simulink model "sim_dinamica_completa_pd"  (R2019b)
settings: Solver=VariableStepAuto  StartTime=0.0  StopTime=10  FixedStep=0.01  RelTol=1e-6
values from neighbouring files (symbols this model uses):
  Kd = [Kp1*Td1 0;         0       Kp2*Td2]    [control_pd_g.m]
  Kp = [Kp1 0;         0   Kp2]    [control_pd_g.m]
  q0 = [90*pi/180;0;0;0]    [control_pd_g.m]
  q_ = [110*pi/180;-30*pi/180;0;0]    [control_pd_g.m]
  theta = load('../theta.mat').theta    [control_pd_g.m]    (also in modelo_dinamico_lineal.m)
settings Model: Creator=AlejnadroZapett  LastModifiedBy=AlejnadroZapett

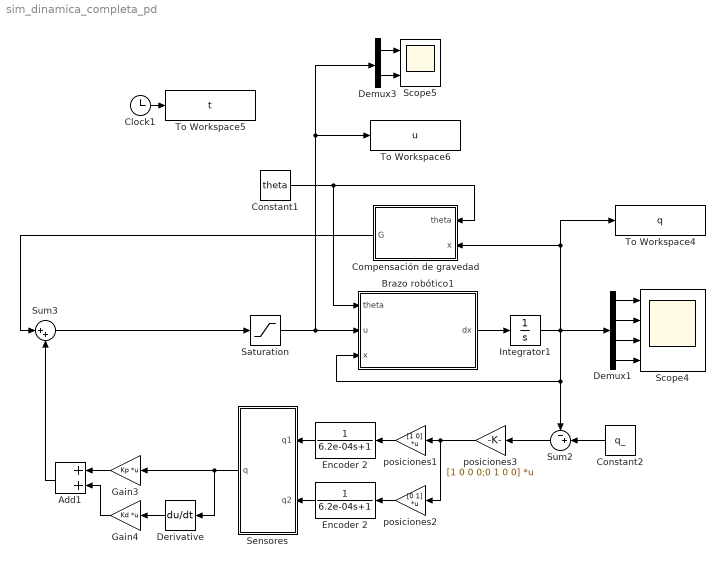
== system sim_dinamica_completa_pd ==
  " Encoder 2 " : TransferFcn  Denominator=[6.2e-04 1]
  Add1 : Sum
  Brazo robótico1 : MATLAB Function  TreatAsAtomicUnit=on
  Clock1 : Clock
  Compensación de gravedad : MATLAB Function  TreatAsAtomicUnit=on
  Constant1 : Constant  Value=theta
  Constant2 : Constant  Value=q_
  Demux1 : Demux
  Demux3 : Demux  Outputs=2
  Derivative : Derivative
  Encoder 2 : TransferFcn  Denominator=[6.2e-04 1]
  Gain3 : Gain  Gain=Kp  Multiplication=Matrix(K*u) (u vector)
  Gain4 : Gain  Gain=Kd  Multiplication=Matrix(K*u) (u vector)
  Integrator1 : Integrator  InitialCondition=q0
  Saturation : Saturate  UpperLimit=255  LowerLimit=-255
  Scope4 : Scope  NumInputPorts=4
  Scope5 : Scope  NumInputPorts=2
  Sensores : MATLAB Function  TreatAsAtomicUnit=on
  Sum2 : Sum  Inputs=-+|
  Sum3 : Sum  Inputs=|++
  To Workspace4 : ToWorkspace  VariableName=q  SampleTime=-1
  To Workspace5 : ToWorkspace  VariableName=t  SampleTime=-1
  To Workspace6 : ToWorkspace  VariableName=u  SampleTime=-1
  posiciones1 : Gain  Gain=[1 0]  Multiplication=Matrix(K*u) (u vector)
  posiciones2 : Gain  Gain=[0 1]  Multiplication=Matrix(K*u) (u vector)
  posiciones3 : Gain  Gain=[1 0 0 0;0 1 0 0]  Multiplication=Matrix(K*u) (u vector)
  wires:
  posiciones2/1 -> Encoder 2/1
  posiciones1/1 -> " Encoder 2 "/1
  Sum2/1 -> posiciones3/1
  Add1/1 -> Sum3/2
  Demux1/4 -> Scope4/4
  Constant2/1 -> Sum2/2
  Demux3/1 -> Scope5/1
  Demux1/2 -> Scope4/2
  Demux1/3 -> Scope4/3
  Saturation/1 -> Brazo robótico1/2(u), To Workspace6/1, Demux3/1
  Demux1/1 -> Scope4/1
  Clock1/1 -> To Workspace5/1
  Constant1/1 -> Compensación de gravedad/1(theta), Brazo robótico1/1(theta)
  Gain3/1 -> Add1/1
  Demux3/2 -> Scope5/2
  Compensación de gravedad/1(G) -> Sum3/1
  Brazo robótico1/1(dx) -> Integrator1/1
  Gain4/1 -> Add1/2
  " Encoder 2 "/1 -> Sensores/1(q1)
  Encoder 2/1 -> Sensores/2(q2)
  Sensores/1(q) -> Derivative/1, Gain3/1
  posiciones3/1 -> posiciones2/1, posiciones1/1
  Derivative/1 -> Gain4/1
  Sum3/1 -> Saturation/1
  Integrator1/1 -> Compensación de gravedad/2(x), To Workspace4/1, Demux1/1, Sum2/1, Brazo robótico1/3(x)

== matlab function sim_dinamica_completa_pd/Sensores ==
  data: q1 input; q2 input; q output
function q = fcn(q1,q2)

q = zeros(2,1);

q(1) = q1;
q(2) = q2;

== matlab function sim_dinamica_completa_pd/Brazo robótico1 ==
  data: theta input; u input; dx output; x input
function dx = fcn(theta,u,x)

dx = zeros(4,1);

u1 = u(1);
u2 = u(2);

q1 = x(1);
q2 = x(2);
dq1 = x(3);
dq2 = x(4);

M11 = (theta(1) + theta(2)*cos(q1));
M12 = (theta(3) + theta(4)*cos(q2));
M21 = (theta(11) + theta(12)*cos(q2));
M22 = theta(13);

C11 = theta(5)*sin(q2)*dq2;
C12 = theta(6)*sin(q2)*dq2;
C21 = theta(14)*sin(q2)*dq1;
C22 = 0;

G1 = theta(7)*cos(q1)+theta(8)*cos(q1+q2);
G2 = theta(14)*cos(q1+q2);

% F1 = theta(9)*dq1 + theta(10)*sign(dq1);
% F2 = theta(16)*dq2 + theta(17)*sign(dq2);
F1 = theta(9)*dq1;
F2 = theta(16)*dq2;

M = [M11 M12;M21 M22];
C = [C11 C12;C21 C22];
G = [G1;G2];
F = [F1;F2];
T = [u1;u2];

D = -inv(M)*(C*[dq1;dq2]+G+F-T);

dx(1) = dq1;
dx(2) = dq2;
dx(3) = D(1);
dx(4) = D(2);

== matlab function sim_dinamica_completa_pd/Compensación de gravedad ==
  data: theta input; G output; x input
function G = fcn(theta,x)

q1 = x(1);
q2 = x(2);

G1 = theta(7)*cos(q1)+theta(8)*cos(q1+q2);
G2 = theta(14)*cos(q1+q2);

G = [G1;G2];
